simulink model "dspsacomp"  (Simulink 6.5)
settings: Solver=FixedStepDiscrete  StartTime=0.0  StopTime=inf  RelTol=1e-3  AbsTol=1e-6
undefined symbols (not defined in the file or in its folder): dfilt
libraries: dspspect3 x4, dsparch4 x1, dspsnks4 x1, dspsrcs4 x1
settings Model: RequirementInfo=9  Creator=The MathWorks Inc.  LastModifiedBy=Shay  ExtModeTrigMode=oneshot  ExtModeArmWhenConnect=off  ExtModeAutoUpdateStatusClock=off  BufferReuse=off  ProdHWDeviceType=Specified
settings DataIOCC: LimitDataPoints=off  SaveOutput=off  SaveTime=off  SignalLoggingName=sigsOut
settings OptimizationCC: BlockReduction=off  BooleanDataType=off  OptimizeBlockIOStorage=off  BufferReuse=off  ExpressionFolding=off  LocalBlockOutputs=off  RollThreshold=2  BufferReusableBoundary=off
settings DebuggingCC: SolverPrmCheckMsg=none  MultiTaskDSMMsg=warning  MultiTaskCondExecSysMsg=none  IntegerOverflowMsg=none  BusObjectLabelMismatch=none  StrictBusMsg=None
settings HardwareCC: ProdHWDeviceType=Specified
settings RTWCC: IncludeERTFirstTime=on

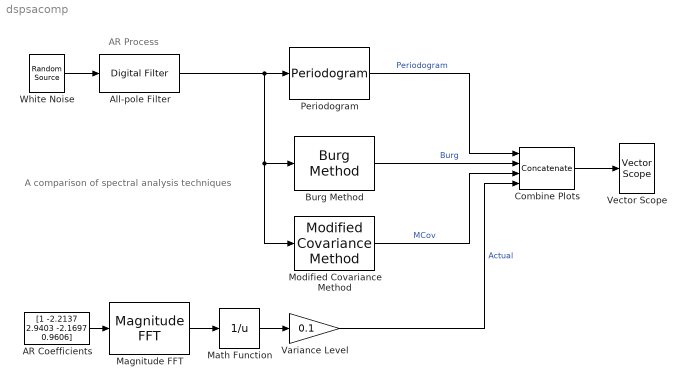
== system dspsacomp ==
  note: A comparison of spectral
      | analysis techniques
  note: AR Process
  AR Coefficients : Constant  Value=[1 -2.2137 2.9403 -2.1697 0.9606]  OutDataType=sfix(16)  ConRadixGroup=Use specified scaling  OutScaling=2^0  SampleTime=inf  FramePeriod=inf
  All-pole Filter : dsparch4/Digital Filter  DialogController=dspdialog.DigitalFilter  DialogControllerArgs=DataTag0  TypePopup=IIR (all poles)  IIRFiltStruct=Direct form II transposed  AllPoleFiltStruct=Direct form  FIRFiltStruct=Direct form  CoeffSource=Specify via dialog  NumCoeffs=[1 2]  DenCoeffs=[1 -2.2137 2.9403 -2.1697 0.9606]  BiQuadCoeffs=[1 0.3 0.4 1 0.1 0.2]  LatticeCoeffs=[0.2 0.4]  denIgnore=on  FiltPerSampPopup=One filter per frame  IC=0  ICnum=0  ICden=0  roundingMode=Floor  overflowMode=off  ScaleValues=1  scaleValueFracLength=14  stageInFracLength=15  stageOutFracLength=15  FilterSource=Specify via dialog  dfiltObjectName=dfilt.dffir([1 2 1])
  Burg Method : dspspect3/Burg Method  SystemSampleTime=-1  inheritOrd=off  ord=4  inheritFFT=off  fftsize=128
  Combine Plots : Concatenate  NumInputs=4  Mode=Horizontal matrix concatenation
  Magnitude FFT : dspspect3/Magnitude FFT  SystemSampleTime=-1  mag_or_magsq=Magnitude squared  fftLenInherit=off  fftsize=128
  Math Function : Math  Operator=reciprocal  SaturateOnIntegerOverflow=on
  Modified Covariance Method : dspspect3/Modified Covariance Method  SystemSampleTime=-1  ord=4  inheritFFT=off  fftsize=128
  Periodogram : dspspect3/Periodogram  SystemSampleTime=-1  wintype=Hamming  Rs=50  beta=5  winsamp=Symmetric  inheritFFT=off  fftsize=128  navg=4
  Variance Level : Gain  Gain=0.1  SaturateOnIntegerOverflow=on
  Vector Scope : dspsnks4/Vector Scope  DialogController=dspdialog.VectorScope  DialogControllerArgs=DataTag1  ScopeProperties=off  Domain=Frequency  HorizSpan=1  DisplayProperties=off  AxisGrid=on  Memory=off  FrameNumber=on  AxisLegend=on  AxisZoom=off  OpenScopeAtSimStart=on  OpenScopeImmediately=off  FigPos=[38 195 560 293]  AxisProperties=on  XUnits=Hertz  XRange=[0...Fs/2]  InheritXIncr=off  XIncr=1/1000  XLabel=Samples  YUnits=dB  YLabel=Amplitude  LineProperties=off  LineColors=[1 0 0]|[0 1 0]|[0 0 1]
      settings: YMin=-36.5241171110829  YMax=35.1414095795369
  White Noise : dspsrcs4/Random Source  SrcType=Gaussian  NormMethod=Ziggurat  CltLength=12  MinVal=0  MaxVal=1  MeanVal=0  VarVal=0.1  RepMode=Specify seed  rawSeed=0  IsInherit=off  SampMode=Discrete  SampTime=1/1000  SampFrame=64  DataType=Double  OutComplex=Real
  wires:
  White Noise/1 -> All-pole Filter/1
  Magnitude FFT/1 -> Math Function/1
  AR Coefficients/1 -> Magnitude FFT/1
  All-pole Filter/1 -> Periodogram/1, Burg Method/1, Modified Covariance Method/1
  Math Function/1 -> Variance Level/1
  Periodogram/1 -> Combine Plots/1  "Periodogram"
  Modified Covariance Method/1 -> Combine Plots/3  "MCov"
  Burg Method/1 -> Combine Plots/2  "Burg"
  Variance Level/1 -> Combine Plots/4  "Actual"
  Combine Plots/1 -> Vector Scope/1
